simulink model "uorb_read_barometer"  (R2018b)
settings: Solver=FixedStepAuto  StartTime=0.0  StopTime=inf  RelTol=1e-3  EnableMultiTasking=on
libraries: px4uORBlib x3
settings Model: SimulationMode=external  ExtModeTrigDuration=10  Creator=Tejas Rajopadhye  LastModifiedBy=Tejas Rajopadhye
settings SolverCC: PositivePriorityOrder=on
settings OptimizationCC: EnhancedBackFolding=on  PassReuseOutputArgsAs=Individual arguments  MaxStackSize=64  OptimizeBlockOrder=speed  DifferentSizesBufferReuse=on  OptimizationCustomize=off
settings DebuggingCC: ParameterTunabilityLossMsg=error
settings HardwareCC: ProdBitPerPointer=32  ProdBitPerSizeT=32  ProdBitPerPtrDiffT=32  ProdLargestAtomicInteger=Long  ProdLargestAtomicFloat=Double  ProdWordSize=32  ProdLongLongMode=on  ProdHWDeviceType=ARM Compatible->ARM Cortex
settings SFSimCC: MATLABDynamicMemAlloc=off
settings RTWCC: SystemTargetFile=ert.tlc  HardwareBoard=PX4 Pixhawk 4  TLCOptions="-aInlineSetEventsForThisBaseRateFcn=TLC_FALSE -aSuppressMultiTaskScheduler=TLC_FALSE  -aRateBasedStepFcn=0"  TemplateMakefile=ert_default_tmf  GenerateReport=on  Toolchain=GNU Tools for PX4 Autopilots  IncludeHyperlinkInReport=on  LaunchReport=on  TargetLang=C++  GenerateTraceInfo=on  GenerateTraceReport=on  GenerateTraceReportSl=on  GenerateTraceReportSf=on  GenerateTraceReportEml=on
settings CodeAppCC: ForceParamTrailComments=on  IgnoreCustomStorageClasses=off  OperatorAnnotations=on  SimulinkDataObjDesc=on  SFDataObjDesc=on  InsertBlockDesc=on

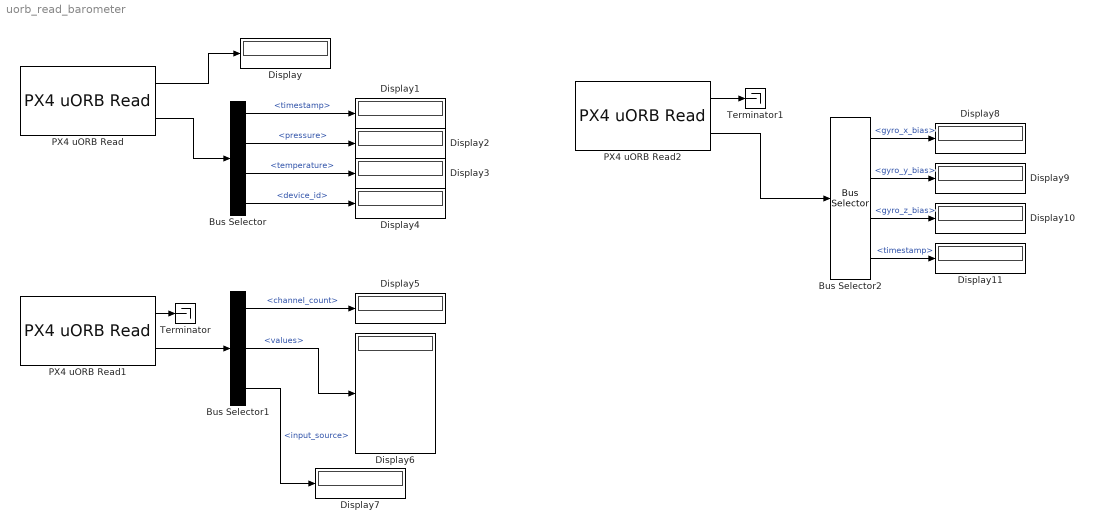
== system uorb_read_barometer ==
  Bus Selector : BusSelector  OutputSignals=timestamp,pressure,temperature,device_id
  Bus Selector1 : BusSelector  OutputSignals=channel_count,values,input_source
  Bus Selector2 : BusSelector  OutputSignals=gyro_x_bias,gyro_y_bias,gyro_z_bias,timestamp
  Display{,1..11} (12 alike) : Display
  PX4 uORB Read : px4uORBlib/PX4 uORB Read  uORBTopic=sensor_baro  sampleTime=-1  BlockingMode=off  BlockTimeout=1e-3
      settings: SourceProductName=Embedded Coder Support Package for PX4 Autopilots
  PX4 uORB Read1 : px4uORBlib/PX4 uORB Read  uORBTopic=input_rc  sampleTime=-1  BlockingMode=off  BlockTimeout=1e-3
      settings: SourceProductName=Embedded Coder Support Package for PX4 Autopilots
  PX4 uORB Read2 : px4uORBlib/PX4 uORB Read  uORBTopic=sensor_bias  sampleTime=-1  BlockingMode=off  BlockTimeout=1e-3
      settings: SourceProductName=Embedded Coder Support Package for PX4 Autopilots
  Terminator : Terminator
  Terminator1 : Terminator
  wires:
  PX4 uORB Read/2 -> Bus Selector/1
  PX4 uORB Read/1 -> Display/1
  Bus Selector/1 -> Display1/1  "<timestamp>"
  Bus Selector/2 -> Display2/1  "<pressure>"
  Bus Selector/3 -> Display3/1  "<temperature>"
  Bus Selector/4 -> Display4/1  "<device_id>"
  PX4 uORB Read1/2 -> Bus Selector1/1
  PX4 uORB Read1/1 -> Terminator/1
  Bus Selector1/1 -> Display5/1  "<channel_count>"
  Bus Selector1/2 -> Display6/1  "<values>"
  Bus Selector1/3 -> Display7/1  "<input_source>"
  PX4 uORB Read2/1 -> Terminator1/1
  PX4 uORB Read2/2 -> Bus Selector2/1
  Bus Selector2/1 -> Display8/1  "<gyro_x_bias>"
  Bus Selector2/2 -> Display9/1  "<gyro_y_bias>"
  Bus Selector2/3 -> Display10/1  "<gyro_z_bias>"
  Bus Selector2/4 -> Display11/1  "<timestamp>"
